simulink model "ch6example6"  (Simulink 5.0)
settings: Solver=FixedStepDiscrete  StartTime=0.0  StopTime=10.0  FixedStep=1/8000  RelTol=1e-3
libraries: commutil2 x1
settings Model: LastModifiedBy=shaoyubin

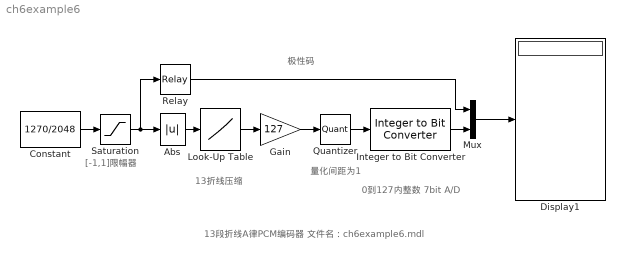
== system ch6example6 ==
  note: 13段折线A律PCM编码器
      | 文件名：ch6example6.mdl
  note: 0到127内整数
      | 7bit A/D
  note: [-1,1]限幅器
  note: 极性码
  note: 13折线压缩
  note: 量化间距为1
  Abs : Abs  SaturateOnIntegerOverflow=on
  Constant : Constant  Value=1270/2048
  Display1 : Display
  Gain : Gain  Gain=127  SaturateOnIntegerOverflow=on
  Integer to Bit Converter : commutil2/Integer to Bit Converter  nbits=7
  Look-Up Table : Lookup  InputValues=[0,1/128,1/64,1/32,1/16,1/8,1/4,1/2,1]  OutputValues=[0:1/8:1]  SaturateOnIntegerOverflow=on
  Mux : Mux  Inputs=2
  Quantizer : Quantizer  QuantizationInterval=1
  Relay : Relay
  Saturation : Saturate  UpperLimit=1  LowerLimit=-1
  wires:
  Constant/1 -> Saturation/1
  Look-Up Table/1 -> Gain/1
  Quantizer/1 -> Integer to Bit Converter/1
  Gain/1 -> Quantizer/1
  Abs/1 -> Look-Up Table/1
  Relay/1 -> Mux/1
  Integer to Bit Converter/1 -> Mux/2
  Mux/1 -> Display1/1
  Saturation/1 -> Abs/1, Relay/1
